simulink model "AMB_L_8_vRTHS_simulation"  (R2021a)
settings: Solver=ode4  StartTime=0.0  StopTime=ttotal  FixedStep=dtsim  RelTol=1e-3
values from neighbouring files (symbols this model uses):
  a1_b0 = 2.13e13    (= 21300000000000)    [AMB_L_1_vRTHS.m]
  a2 = 4.23e6    (= 4230000)    [AMB_L_1_vRTHS.m]
  a3 = 3.3+1.3*randn(1,1)*inc    [AMB_L_1_vRTHS.m]    (also in AMB_L_2_calibration.m = 3.3)
  adaptivegain = diag(10.^[8.4 6.2 2.1 0.8])    [AMB_L_1_vRTHS.m]    (also in AMB_L_2_calibration.m = gain2; AMB_L_5_optimization.m = diag(10.^op_location'); AMB_L_6_R2function.m = diag(10.^x); AMB_L_7_J2andInputs.m = diag(10.^x))
  Ar = [zeros(3),eye(3);-M\K -M\C]    [AMB_L_1_vRTHS.m]
  b1 = 425+3.3*randn(1,1)*inc    [AMB_L_1_vRTHS.m]    (also in AMB_L_2_calibration.m = 425)
  b2 = 1e5+3.3e3*randn(1,1)*inc    [AMB_L_1_vRTHS.m]    (also in AMB_L_2_calibration.m = 100000)
  Br = [zeros(3,1);-ones(3,1)]    [AMB_L_1_vRTHS.m]
  Cr = eye(6)    [AMB_L_1_vRTHS.m]
  Derivadas = [u;dudt;dudt2;dudt3]    [AMB_L_1_vRTHS.m]
  Dr = zeros(6,1)    [AMB_L_1_vRTHS.m]
  dtsim = 1/fs    (= 0.000244140625)    [AMB_L_1_vRTHS.m]
  gain = 1    [AMB_L_1_vRTHS.m]
  max_amb = [amb0max,amb1max,amb2max,amb3max]    [AMB_L_1_vRTHS.m]
  min_amb = [amb0min,amb1min,amb2min,amb3min]    [AMB_L_1_vRTHS.m]
  rms_noise_desp = 6.25e-14    [AMB_L_1_vRTHS.m]
  rms_noise_F = 1.16e-3    (= 0.00116)    [AMB_L_1_vRTHS.m]
  sat_limit_lower = -3.8    [AMB_L_1_vRTHS.m]
  sat_limit_upper = +3.8    (= 3.8)    [AMB_L_1_vRTHS.m]
  ssAe = [0,1;-ke/me,-ce/me]    [AMB_L_1_vRTHS.m]
  ssAn = [zeros(3),eye(3);-Mn\Kn,-Mn\Cn]    [AMB_L_1_vRTHS.m]
  ssBe = [0;1/me]    [AMB_L_1_vRTHS.m]
  ssBn = [zeros(3,2);-Mn\M*G1,-Mn\G2]    [AMB_L_1_vRTHS.m]
  ssCe = [1,0;0,1]    [AMB_L_1_vRTHS.m]
  ssCn = [eye(3),zeros(3)]    [AMB_L_1_vRTHS.m]
  ssDe = [0;0]    [AMB_L_1_vRTHS.m]
  ssDn = zeros(3,2)    [AMB_L_1_vRTHS.m]
undefined symbols (not defined in the file or in its folder): denfilter, numfilter
libraries: simulink x2
settings Model: Creator=cristobal  LastModifiedBy=MSI
settings SolverCC: AlgebraicLoopSolver=TrustRegion
settings DataIOCC: ReturnWorkspaceOutputs=off
settings DebuggingCC: SFMachineParentedDataDiag=warning  ArithmeticOperatorsInVariantConditions=warning
settings SFSimCC: SimUseLocalCustomCode=off  CustomCodeUndefinedFunction=UseInterfaceOnly
settings RTWCC: RTWUseLocalCustomCode=off
settings CodeAppCC: StateflowObjectComments=on

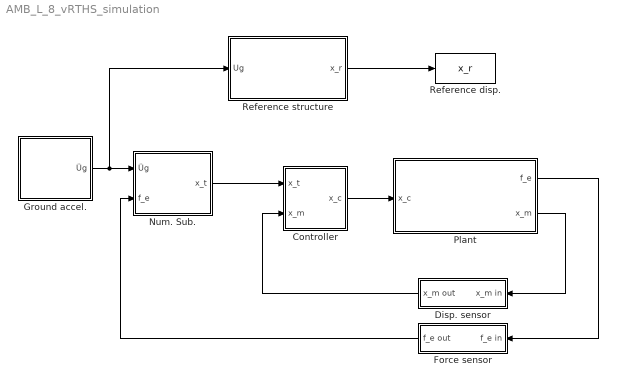
== system AMB_L_8_vRTHS_simulation ==
  Controller : Subsystem
  Disp. sensor : Subsystem
  Force sensor : Subsystem
  Ground accel. : Subsystem
  Num. Sub. : Subsystem
  Plant : Subsystem
  Reference disp. : ToWorkspace  VariableName=x_r  SaveFormat=Timeseries  SampleTime=-1
  Reference structure : Subsystem
  wires:
  Num. Sub./1(x_t) -> Controller/1(x_t)
  Controller/1(x_c) -> Plant/1(x_c)
  Plant/1(f_e) -> Force sensor/1(f_e in)
  Plant/2(x_m) -> Disp. sensor/1(x_m in)
  Ground accel./1(Üg) -> Num. Sub./1(Üg), Reference structure/1(Ug)
  Reference structure/1(x_r) -> Reference disp./1
  Disp. sensor/1(x_m out) -> Controller/2(x_m)
  Force sensor/1(f_e out) -> Num. Sub./2(f_e)

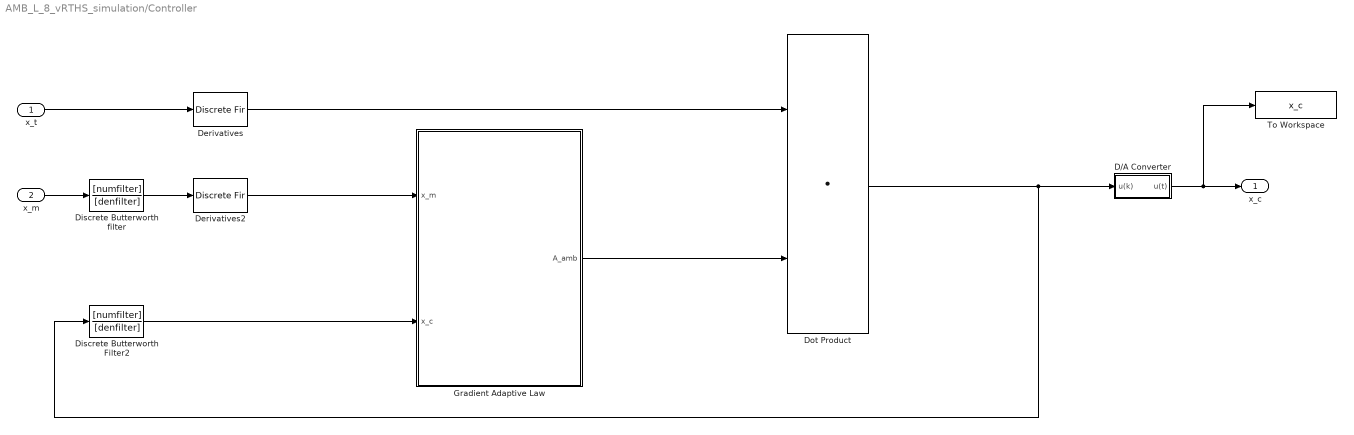
== system AMB_L_8_vRTHS_simulation/Controller ==
  x_t : Inport
  x_m : Inport  Port=2
  D/A Converter : Subsystem
  Derivatives : DiscreteFir  Coefficients=Derivadas
  Derivatives2 : DiscreteFir  Coefficients=Derivadas
  Discrete Butterworth Filter2 : DiscreteTransferFcn  Numerator=[numfilter]  Denominator=[denfilter]
  Discrete Butterworth filter : DiscreteTransferFcn  Numerator=[numfilter]  Denominator=[denfilter]
  Dot Product : DotProduct  InputSameDT=on  OutDataTypeStr=Inherit: Inherit via internal rule
  Gradient Adaptive Law : Subsystem
  To Workspace : ToWorkspace  VariableName=x_c  SaveFormat=Timeseries  SampleTime=-1
  x_c : Outport  VectorParamsAs1DForOutWhenUnconnected=off
  wires:
  Derivatives2/1 -> Gradient Adaptive Law/1(x_m)
  Discrete Butterworth Filter2/1 -> Gradient Adaptive Law/2(x_c)
  x_m/1 -> Discrete Butterworth filter/1
  Discrete Butterworth filter/1 -> Derivatives2/1
  x_t/1 -> Derivatives/1
  Dot Product/1 -> D/A Converter/1(u(k)), Discrete Butterworth Filter2/1
  Derivatives/1 -> Dot Product/1
  Gradient Adaptive Law/1(A_amb) -> Dot Product/2
  D/A Converter/1(u(t)) -> To Workspace/1, x_c/1

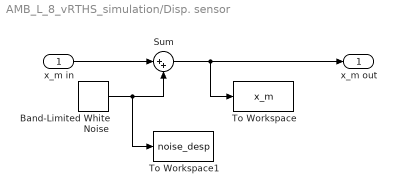
== system AMB_L_8_vRTHS_simulation/Disp. sensor ==
  x_m in : Inport
  Band-Limited White Noise : simulink/Sources/Band-Limited White Noise  Cov=[rms_noise_desp]  Ts=dtsim  seed=ceil(rand(1)*10000)
  Sum : Sum  Inputs=|++
  To Workspace : ToWorkspace  VariableName=x_m  SaveFormat=Timeseries  SampleTime=-1
  To Workspace1 : ToWorkspace  VariableName=noise_desp  SaveFormat=Timeseries  SampleTime=-1
  x_m out : Outport  VectorParamsAs1DForOutWhenUnconnected=off
  wires:
  Band-Limited White Noise/1 -> To Workspace1/1, Sum/2
  Sum/1 -> x_m out/1, To Workspace/1
  x_m in/1 -> Sum/1

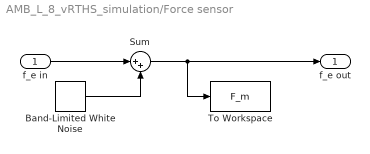
== system AMB_L_8_vRTHS_simulation/Force sensor ==
  f_e in : Inport
  Band-Limited White Noise : simulink/Sources/Band-Limited White Noise  Cov=[rms_noise_F]  Ts=dtsim  seed=ceil(rand(1)*20000)
  Sum : Sum  Inputs=|++
  To Workspace : ToWorkspace  VariableName=F_m  SaveFormat=Timeseries  SampleTime=-1
  f_e out : Outport  VectorParamsAs1DForOutWhenUnconnected=off
  wires:
  f_e in/1 -> Sum/1
  Sum/1 -> To Workspace/1, f_e out/1
  Band-Limited White Noise/1 -> Sum/2

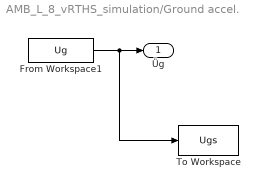
== system AMB_L_8_vRTHS_simulation/Ground accel. ==
  From Workspace1 : FromWorkspace  VariableName=Ug  OutputAfterFinalValue=Setting to zero
  To Workspace : ToWorkspace  VariableName=Ugs  SaveFormat=Timeseries  SampleTime=-1
  Üg : Outport  VectorParamsAs1DForOutWhenUnconnected=off
  wires:
  From Workspace1/1 -> To Workspace/1, Üg/1

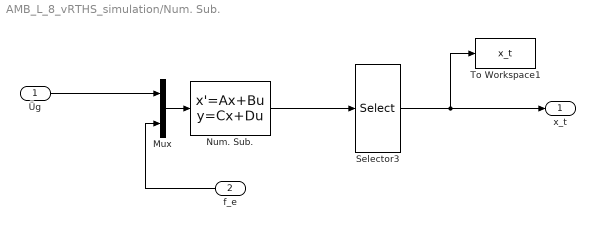
== system AMB_L_8_vRTHS_simulation/Num. Sub. ==
  Üg : Inport
  f_e : Inport  Port=2
  Mux : Mux  Inputs=2
  Num. Sub. : StateSpace  A=ssAn  B=ssBn  C=ssCn  D=ssDn  InitialCondition=0
  Selector3 : Selector  InputPortWidth=3  IndexOptions=Index vector (dialog)  Indices=[1]  OutputSizes=1
  To Workspace1 : ToWorkspace  VariableName=x_t  SaveFormat=Timeseries  SampleTime=-1
  x_t : Outport  VectorParamsAs1DForOutWhenUnconnected=off
  wires:
  Mux/1 -> Num. Sub./1
  Selector3/1 -> x_t/1, To Workspace1/1
  Üg/1 -> Mux/1
  Num. Sub./1 -> Selector3/1
  f_e/1 -> Mux/2

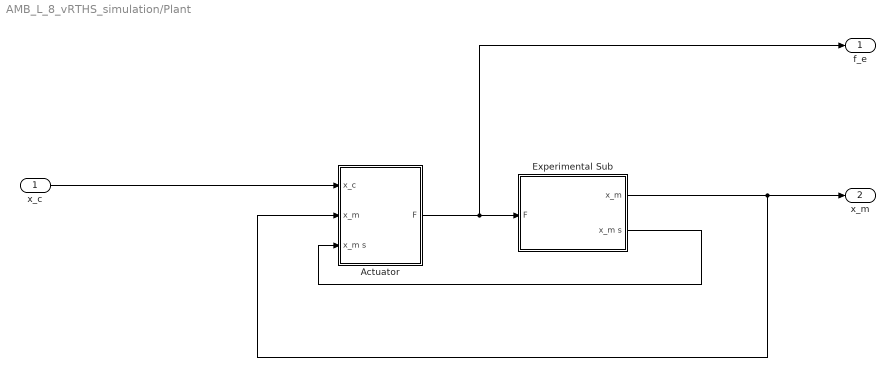
== system AMB_L_8_vRTHS_simulation/Plant ==
  x_c : Inport
  Actuator : Subsystem
  Experimental Sub : Subsystem
  f_e : Outport  VectorParamsAs1DForOutWhenUnconnected=off
  x_m : Outport  Port=2  VectorParamsAs1DForOutWhenUnconnected=off
  wires:
  Actuator/1(F) -> f_e/1, Experimental Sub/1(F)
  x_c/1 -> Actuator/1(x_c)
  Experimental Sub/2(x_m s) -> Actuator/3(x_m s)
  Experimental Sub/1(x_m) -> x_m/1, Actuator/2(x_m)

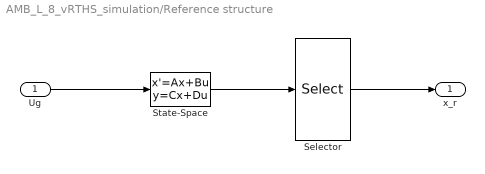
== system AMB_L_8_vRTHS_simulation/Reference structure ==
  Ug : Inport
  Selector : Selector  InputPortWidth=6  IndexOptions=Index vector (dialog)  Indices=[1]  OutputSizes=1
  State-Space : StateSpace  A=Ar  B=Br  C=Cr  D=Dr  InitialCondition=0
  x_r : Outport  VectorParamsAs1DForOutWhenUnconnected=off
  wires:
  State-Space/1 -> Selector/1
  Selector/1 -> x_r/1
  Ug/1 -> State-Space/1

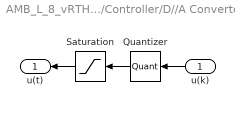
== system AMB_L_8_vRTHS_simulation/Controller/D//A Converter ==
  u(k) : Inport
  Quantizer : Quantizer  QuantizationInterval=quantize_int
  Saturation : Saturate  UpperLimit=sat_limit_upper  LowerLimit=sat_limit_lower
  u(t) : Outport  VectorParamsAs1DForOutWhenUnconnected=off
  wires:
  Saturation/1 -> u(t)/1
  Quantizer/1 -> Saturation/1
  u(k)/1 -> Quantizer/1

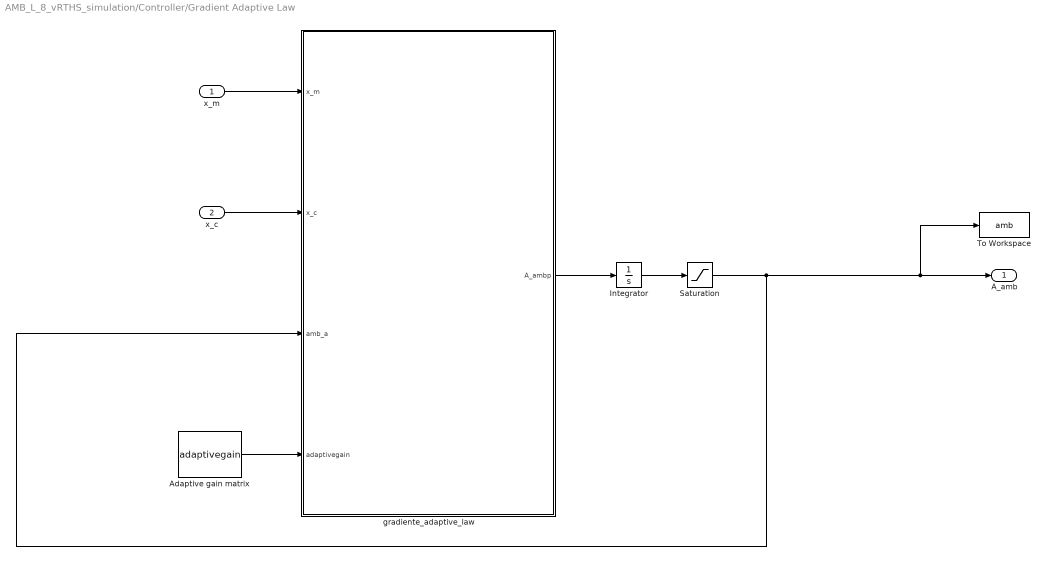
== system AMB_L_8_vRTHS_simulation/Controller/Gradient Adaptive Law ==
  x_m : Inport
  x_c : Inport  Port=2
  Adaptive gain matrix : Constant  Value=adaptivegain
  Integrator : Integrator  InitialCondition=A_amb_i'
  Saturation : Saturate  UpperLimit=[max_amb]  LowerLimit=min_amb
  To Workspace : ToWorkspace  VariableName=amb  SaveFormat=Timeseries  SampleTime=-1
  gradiente_adaptive_law : MATLAB Function  TreatAsAtomicUnit=on
  A_amb : Outport  VectorParamsAs1DForOutWhenUnconnected=off
  wires:
  Integrator/1 -> Saturation/1
  x_c/1 -> gradiente_adaptive_law/2(x_c)
  Adaptive gain matrix/1 -> gradiente_adaptive_law/4(adaptivegain)
  gradiente_adaptive_law/1(A_ambp) -> Integrator/1
  x_m/1 -> gradiente_adaptive_law/1(x_m)
  Saturation/1 -> To Workspace/1, A_amb/1, gradiente_adaptive_law/3(amb_a)

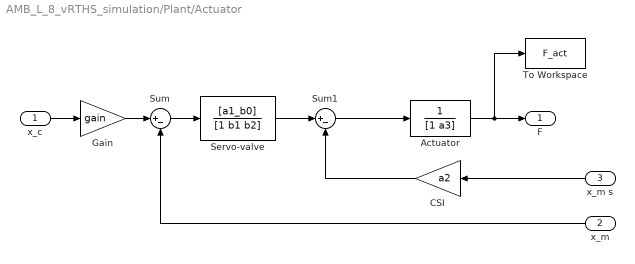
== system AMB_L_8_vRTHS_simulation/Plant/Actuator ==
  x_c : Inport
  x_m : Inport  Port=2
  x_m s : Inport  Port=3
  Actuator : TransferFcn  Denominator=[1 a3]
  CSI : Gain  Gain=a2
  Gain : Gain  Gain=gain
  Servo-valve : TransferFcn  Numerator=[a1_b0]  Denominator=[1 b1 b2]
  Sum : Sum  Inputs=|+-
  Sum1 : Sum  Inputs=|+-
  To Workspace : ToWorkspace  VariableName=F_act  SaveFormat=Timeseries  SampleTime=-1
  F : Outport  VectorParamsAs1DForOutWhenUnconnected=off
  wires:
  CSI/1 -> Sum1/2
  Actuator/1 -> To Workspace/1, F/1
  Sum1/1 -> Actuator/1
  Sum/1 -> Servo-valve/1
  Servo-valve/1 -> Sum1/1
  x_c/1 -> Gain/1
  Gain/1 -> Sum/1
  x_m/1 -> Sum/2
  x_m s/1 -> CSI/1

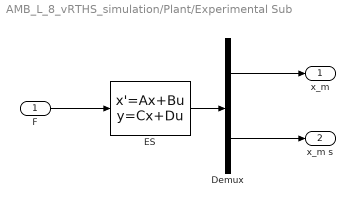
== system AMB_L_8_vRTHS_simulation/Plant/Experimental Sub ==
  F : Inport
  Demux : Demux  Outputs=2
  ES : StateSpace  A=ssAe  B=ssBe  C=ssCe  D=ssDe  InitialCondition=0
  x_m : Outport  VectorParamsAs1DForOutWhenUnconnected=off
  x_m s : Outport  Port=2  VectorParamsAs1DForOutWhenUnconnected=off
  wires:
  ES/1 -> Demux/1
  F/1 -> ES/1
  Demux/2 -> x_m s/1
  Demux/1 -> x_m/1

== matlab function AMB_L_8_vRTHS_simulation/Controller/Gradient Adaptive Law/gradiente_adaptive_law ==
  data: x_m input; x_c input; amb_a input; A_ambp output; adaptivegain input
function A_ambp   = fcn(x_m,x_c,amb_a,adaptivegain)
error=(x_c-amb_a'*x_m)/(1+(x_m'*x_m));
A_ambp=adaptivegain*error*x_m;
